simulink model "Current_torque_111"  (R2017b)
settings: Solver=ode45  StartTime=0.0  StopTime=3  MaxStep=1e-4  RelTol=1e-3  EnableMultiTasking=on
libraries: neural x38, fuzblock x6, simulink x1
(part 2 of 3)

== system Current_torque_111/CNN/Layer 5 ==
  "a{4} " : Inport  PortDimensions=5
      mask Display: e = 0.06;c1 = [120 230 180]/255;c2 = ([120 230 180]+0)/(256+128);c3 = ([120 230 180]+128)/(256+128);patch([0 1 1 0],[0 0 1 1],c1);patch([0 1 1 1-e 1-e 0+e],[0 0 1 1-e 0+e 0+e],c2);patch([0 0 1 1-e 0+e 0+e],[0 1 1 1-e 1-e 0+e],c3);plot([0 1 1 0 0],[0 0 1 1 0]);
  Delays 1 : Subsystem
      mask Display: e = 0.06;c1 = [120 150 230]/255;c2 = ([120 150 230]+0)/383;c3 = ([120 150 230]+128)/383;patch([0 1 1 0],[0 0 1 1],c1);patch([0 1 1 1-e 1-e 0+e],[0 0 1 1-e 0+e 0+e],c2);patch([0 0 1 1-e 0+e 0+e],[0 1 1 1-e 1-e 0+e],c3);plot([0 1 1 0 0],[0 0 1 1 0]);disp('0');
  "LW{5,4}" : Subsystem
      mask Display: e = 0.06;c1 = [120 150 230]/255;c2 = ([120 150 230]+0)/383;c3 = ([120 150 230]+128)/383;patch([0 1 1 0],[0 0 1 1],c1);patch([0 1 1 1-e 1-e 0+e],[0 0 1 1-e 0+e 0+e],c2);patch([0 0 1 1-e 0+e 0+e],[0 1 1 1-e 1-e 0+e],c3);plot([0 1 1 0 0],[0 0 1 1 0]);disp('W');
  "b{5}" : Constant  Value=-0.12962536607997010573711804681806825101375579833984375
      mask Display: e = 0.06;c1 = [120 150 230]/255;c2 = ([120 150 230]+0)/383;c3 = ([120 150 230]+128)/383;patch([0 1 1 0],[0 0 1 1],c1);patch([0 1 1 1-e 1-e 0+e],[0 0 1 1-e 0+e 0+e],c2);patch([0 0 1 1-e 0+e 0+e],[0 1 1 1-e 1-e 0+e],c3);plot([0 1 1 0 0],[0 0 1 1 0]);disp('b');
  netsum : Sum  Inputs=2  SaturateOnIntegerOverflow=on  InputSameDT=on  OutDataTypeStr=Inherit: Same as first input
      mask Display: e = 0.06;c1 = [120 150 230]/255;c2 = ([120 150 230]+0)/383;c3 = ([120 150 230]+128)/383;patch([0 1 1 0],[0 0 1 1],c1);patch([0 1 1 1-e 1-e 0+e],[0 0 1 1-e 0+e 0+e],c2);patch([0 0 1 1-e 0+e 0+e],[0 1 1 1-e 1-e 0+e],c3);plot([0 1 1 0 0],[0 0 1 1 0]);disp('+');
  purelin : neural/Transfer Functions/purelin
  "a{5}" : Outport  InitialOutput=0
      mask Display: e = 0.06;c1 = [120 230 180]/255;c2 = ([120 230 180]+0)/(256+128);c3 = ([120 230 180]+128)/(256+128);patch([0 1 1 0],[0 0 1 1],c1);patch([0 1 1 1-e 1-e 0+e],[0 0 1 1-e 0+e 0+e],c2);patch([0 0 1 1-e 0+e 0+e],[0 1 1 1-e 1-e 0+e],c3);plot([0 1 1 0 0],[0 0 1 1 0]);
  wires:
  purelin/1 -> "a{5}"/1
  netsum/1 -> purelin/1
  "b{5}"/1 -> netsum/2
  "LW{5,4}"/1("lz{5,4}") -> netsum/1
  Delays 1/1("pd{5,4}") -> "LW{5,4}"/1("ad{5,4}")
  "a{4} "/1 -> Delays 1/1("p{5}")

== system Current_torque_111/CNN/Process Input 1 ==
  x : Inport  PortDimensions=2
      mask Display: e = 0.06;c1 = [120 230 180]/255;c2 = ([120 230 180]+0)/(256+128);c3 = ([120 230 180]+128)/(256+128);patch([0 1 1 0],[0 0 1 1],c1);patch([0 1 1 1-e 1-e 0+e],[0 0 1 1-e 0+e 0+e],c2);patch([0 0 1 1-e 0+e 0+e],[0 1 1 1-e 1-e 0+e],c3);plot([0 1 1 0 0],[0 0 1 1 0]);
  mapminmax : neural/Processing Functions/mapminmax  xmin=[-120;1.5]  xmax=[-1;120]  ymin=-1  ymax=1
  p : Outport  PortDimensions=2
      mask Display: e = 0.06;c1 = [120 230 180]/255;c2 = ([120 230 180]+0)/(256+128);c3 = ([120 230 180]+128)/(256+128);patch([0 1 1 0],[0 0 1 1],c1);patch([0 1 1 1-e 1-e 0+e],[0 0 1 1-e 0+e 0+e],c2);patch([0 0 1 1-e 0+e 0+e],[0 1 1 1-e 1-e 0+e],c3);plot([0 1 1 0 0],[0 0 1 1 0]);
  wires:
  mapminmax/1 -> p/1
  x/1 -> mapminmax/1

== system Current_torque_111/CNN/Process Output 1 ==
  a : Inport  PortDimensions=1
      mask Display: e = 0.06;c1 = [120 230 180]/255;c2 = ([120 230 180]+0)/(256+128);c3 = ([120 230 180]+128)/(256+128);patch([0 1 1 0],[0 0 1 1],c1);patch([0 1 1 1-e 1-e 0+e],[0 0 1 1-e 0+e 0+e],c2);patch([0 0 1 1-e 0+e 0+e],[0 1 1 1-e 1-e 0+e],c3);plot([0 1 1 0 0],[0 0 1 1 0]);
  mapminmax_reverse : neural/Processing Functions/mapminmax_reverse  xmin=0.599199999999999954880536279234  xmax=104.359999999999999431565811392  ymin=-1  ymax=1
  y : Outport  PortDimensions=1
      mask Display: e = 0.06;c1 = [120 230 180]/255;c2 = ([120 230 180]+0)/(256+128);c3 = ([120 230 180]+128)/(256+128);patch([0 1 1 0],[0 0 1 1],c1);patch([0 1 1 1-e 1-e 0+e],[0 0 1 1-e 0+e 0+e],c2);patch([0 0 1 1-e 0+e 0+e],[0 1 1 1-e 1-e 0+e],c3);plot([0 1 1 0 0],[0 0 1 1 0]);
  wires:
  mapminmax_reverse/1 -> y/1
  a/1 -> mapminmax_reverse/1

== system Current_torque_111/PI Torque controller/PI-Te-iq ==
  In1 : Inport
  Integrator : Integrator  LimitOutput=on  UpperSaturationLimit=120  LowerSaturationLimit=-120
  Scope1 : Scope
  Scope3 : Scope
  Sum2 : Sum  Inputs=|++  SaturateOnIntegerOverflow=on  InputSameDT=on  OutDataTypeStr=Inherit: Same as first input
  kii : Gain  Gain=Ki  SaturateOnIntegerOverflow=on  OutDataTypeStr=Inherit: Same as input  ParamDataTypeStr=Inherit: Same as input
  kpi : Gain  Gain=Kp  SaturateOnIntegerOverflow=on  OutDataTypeStr=Inherit: Same as input  ParamDataTypeStr=Inherit: Same as input
  limit1 : Saturate  UpperLimit=120  LowerLimit=-120
  iq : Outport
  wires:
  In1/1 -> kpi/1, kii/1
  kpi/1 -> Sum2/1
  kii/1 -> Integrator/1
  Integrator/1 -> Scope1/1, Sum2/2
  Sum2/1 -> limit1/1, Scope3/1
  limit1/1 -> iq/1

== system Current_torque_111/PI current controller/PI-U-d ==
  In1 : Inport
  Integrator : Integrator  LimitOutput=on  UpperSaturationLimit=120  LowerSaturationLimit=-120
  Scope1 : Scope
  Scope3 : Scope
  Sum2 : Sum  Inputs=|++  SaturateOnIntegerOverflow=on  InputSameDT=on  OutDataTypeStr=Inherit: Same as first input
  kii : Gain  Gain=Ki  SaturateOnIntegerOverflow=on  OutDataTypeStr=Inherit: Same as input  ParamDataTypeStr=Inherit: Same as input
  kpi : Gain  Gain=Kp  SaturateOnIntegerOverflow=on  OutDataTypeStr=Inherit: Same as input  ParamDataTypeStr=Inherit: Same as input
  limit1 : Saturate  UpperLimit=120  LowerLimit=-120
  usd* : Outport
  wires:
  limit1/1 -> usd*/1
  Sum2/1 -> Scope3/1, limit1/1
  Integrator/1 -> Sum2/2, Scope1/1
  kii/1 -> Integrator/1
  kpi/1 -> Sum2/1
  In1/1 -> kii/1, kpi/1

== system Current_torque_111/PI current controller/PI-U-q ==
  In1 : Inport
  Integrator : Integrator
  Scope3 : Scope
  Sum2 : Sum  Inputs=|++  SaturateOnIntegerOverflow=on  InputSameDT=on  OutDataTypeStr=Inherit: Same as first input
  kii : Gain  Gain=Ki  SaturateOnIntegerOverflow=on  OutDataTypeStr=Inherit: Same as input  ParamDataTypeStr=Inherit: Same as input
  kpi : Gain  Gain=Kp  SaturateOnIntegerOverflow=on  OutDataTypeStr=Inherit: Same as input  ParamDataTypeStr=Inherit: Same as input
  limit2 : Saturate  UpperLimit=inf  LowerLimit=-inf
  usd* : Outport
  wires:
  limit2/1 -> usd*/1
  Sum2/1 -> Scope3/1, limit2/1
  In1/1 -> kpi/1, kii/1
  kpi/1 -> Sum2/1
  kii/1 -> Integrator/1
  Integrator/1 -> Sum2/2

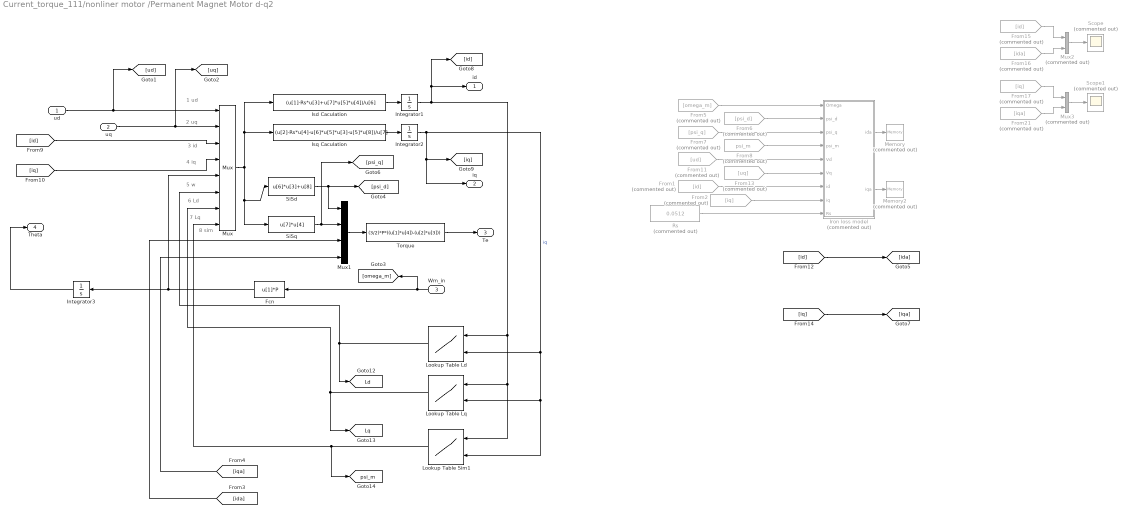
== system Current_torque_111/nonliner motor /Permanent Magnet Motor d-q2 ==
  note: 3 id
  note: 1 ud
  note: 2 uq
  note: 4 iq
  note: 5 w
  note: 6 Ld
  note: 7 Lq
  note: 8 sim
  ud : Inport
  uq : Inport  Port=2
  Wm_in : Inport  Port=3
  Fcn : Fcn  Expr=u[1]*P
  From1 : From  Commented=on  GotoTag=id
  From11 : From  Commented=on  GotoTag=ud
  From13 : From  Commented=on  GotoTag=uq
  From15 : From  Commented=on  GotoTag=id
  From16 : From  Commented=on  GotoTag=ida
  From17 : From  Commented=on  GotoTag=iq
  From2 : From  Commented=on  GotoTag=iq
  From21 : From  Commented=on  GotoTag=iqa
  From5 : From  Commented=on  GotoTag=omega_m
  From6 : From  Commented=on  GotoTag=psi_d
  From7 : From  Commented=on  GotoTag=psi_q
  From8 : From  Commented=on  GotoTag=psi_m  TagVisibility=global
  Integrator1 : Integrator
  Integrator2 : Integrator
  Integrator3 : Integrator
  Iron loss model : Subsystem  Commented=on
  Isd Caculation : Fcn  Expr=(u[1]-Rs*u[3]+u[7]*u[5]*u[4])/u[6]
  Isq Caculation : Fcn  Expr=(u[2]-Rs*u[4]-u[6]*u[5]*u[3]-u[5]*u[8])/u[7]
  Lookup Table Ld : Lookup2D  RowIndex=|  ColumnIndex=|  Table=1e-3*[[0.843,0.842,0.841,0.835,0.822,0.812,0.791,0.763,0.733,0.707,0.683,0.661,0.639];[0.848,0.847,0.846,0.840,0.831,0.814,0.786,0.754,0.723,0.695,0.674,0.651,0.631];[0.852,0.851,0.848,0.844,0.836,0.813,0.777,0.740,0.705,0.682,0.658,0.636,0.618];[0.858,0.857,0.856,0.848,0.831,0.806,0.763,0.727,0.695,0.664,0.643,0.620,0.602];[0.864,0.863,0.860,0.852,0.829,0.796,0.758,0.715,0.682,0.655,0.629,0.607,0.586];[0.870,0.867,0.863,0.850,0.820,0.783,0.748,0.712,0.677,0.650,0.624,0.600,0.580];[0.882,0.875,0.868,0.848,0.808,0.770,0.735,0.707,0.682,0.653,0.621,0.602,0.576];[0.892,0.889,0.873,0.835,0.796,0.757,0.723,0.701,0.678,0.653,0.632,0.603,0.575];[0.902,0.896,0.869,0.819,0.773,0.741,0.712,0.683,0.663,0.646,0.626,0.604,0.584];[0.906,0.892,0.843,0.786,0.750,0.713,0.691,0.662,0.643,0.629,0.611,0.595,0.576];[0.891,0.860,0.798,0.747,0.704,0.685,0.664,0.640,0.615,0.602,0.596,0.576,0.566];[0.838,0.800,0.749,0.707,0.670,0.653,0.628,0.613,0.588,0.576,0.562,0.558,0.546];[0.733,0.700,0.667,0.636,0.612,0.605,0.594,0.579,0.564,0.544,0.529,0.521,0.517]]
      RowIndex=|
      | [-119.9923
      | -109.9929
      | -99.9936
      | -89.9943
      | -79.9949
      | -69.9955
      | -59.9962
      | -49.9968
      | -39.9974
      | -29.9981
      | -19.9987
      | -9.9994
      | 0]
      ColumnIndex=|
      | [0.0000
      | 9.9613
      | 20.0042
      | 29.9654
      | 40.0083
      | 49.9696
      | 60.0125
      | 69.9738
      | 80.0167
      | 89.8146
      | 99.6126
      | 110.2270
      | 120.0250]
  Lookup Table Lq : Lookup2D  RowIndex=|  ColumnIndex=|  Table=1e-3*[[2.7,2.65,2.62,2.45,2.3,2.23,2.1,1.85,1.74,1.61,1.5,1.43,1.33];[2.75,2.7,2.65,2.46,2.31,2.22,2.08,1.84,1.73,1.6,1.49,1.42,1.32];[2.8,2.75,2.7,2.47,2.32,2.21,2.05,1.83,1.72,1.59,1.48,1.4,1.31];[2.9,2.8,2.72,2.48,2.33,2.2,2.02,1.82,1.71,1.58,1.47,1.37,1.3];[2.95,2.85,2.74,2.49,2.34,2.15,2,1.81,1.7,1.57,1.46,1.35,1.29];[3,2.9,2.77,2.5,2.33,2.14,1.95,1.8,1.67,1.56,1.45,1.34,1.28];[3.1,2.95,2.79,2.51,2.32,2.13,1.92,1.79,1.65,1.55,1.44,1.33,1.27];[3.2,3,2.8,2.52,2.3,2.1,1.9,1.75,1.63,1.54,1.43,1.32,1.26];[3.3,3.07,2.78,2.5,2.25,2,1.85,1.72,1.6,1.53,1.4,1.31,1.25];[3.37,3.1,2.75,2.45,2.2,1.99,1.82,1.7,1.55,1.48,1.38,1.3,1.24];[3.4,3.05,2.7,2.4,2.15,1.98,1.8,1.68,1.52,1.46,1.36,1.28,1.23];[3.35,3.02,2.65,2.35,2.1,1.95,1.75,1.65,1.51,1.44,1.35,1.25,1.22];[3.3,3,2.6,2.3,2,1.9,1.7,1.6,1.5,1.4,1.3,1.22,1.2]]
      RowIndex=|
      | [-119.9923
      | -109.9929
      | -99.9936
      | -89.9943
      | -79.9949
      | -69.9955
      | -59.9962
      | -49.9968
      | -39.9974
      | -29.9981
      | -19.9987
      | -9.9994
      | 0]
      ColumnIndex=|
      | [0.0000
      | 9.9613
      | 20.0042
      | 29.9654
      | 40.0083
      | 49.9696
      | 60.0125
      | 69.9738
      | 80.0167
      | 89.8146
      | 99.6126
      | 110.2270
      | 120.0250]
  Lookup Table Sim1 : Lookup2D  RowIndex=|  ColumnIndex=|  Table=1e-3*[[129.6,128.4,127.5,126.5,125.5,124,123,121,119.8,118.2,116.5,114.2,110.3];[129.7,127.2,126.2,125,124,123,122,120,119,117.1,115,112.2,106.4];[130,126.2,125,123.5,122,121,120,118,116,114.7,112,110.5,104.1];[130.4,126.6,123.5,122.2,121,118,117,115,113,112,110,108,101.8];[130.8,127.6,123,120.5,118.9,116.5,113,111,110,108.8,107.5,106,100.4];[131.2,128.2,125.1,118.8,116.3,115,111.6,110,108.9,107,105,104,98.1];[131.9,130,127,118.1,115.0,113.4,110,109,107,104.2,102.8,101.2,96.7];[132.4,130.5,128,119.4,114,113,109.5,108,106,102.9,101.6,100.5,95.1];[132.8,130.6,128.7,120.5,114.5,113.5,110.8,107.5,105.6,101.7,100.5,98.8,94.5];[132.9,130.2,127.9,121,115.5,112.7,110.5,108.5,106.5,103.2,101.5,98.9,92.7];[132.2,129.9,125.9,121.3,115.9,111.5,109.4,107.8,107,102.7,101,97.5,91.1];[131.5,129.0,125.6,120.7,115.3,110.7,109,108,106.6,102.6,99.7,95.9,88.7];[130.8,128.6,124.6,120.5,117.4,111.4,110,109,107.5,103.1,100.4,96.5,88.6]]
      RowIndex=|
      | [-119.9923
      | -109.9929
      | -99.9936
      | -89.9943
      | -79.9949
      | -69.9955
      | -59.9962
      | -49.9968
      | -39.9974
      | -29.9981
      | -19.9987
      | -9.9994
      | 0]
      ColumnIndex=|
      | [0.0000
      | 9.9613
      | 20.0042
      | 29.9654
      | 40.0083
      | 49.9696
      | 60.0125
      | 69.9738
      | 80.0167
      | 89.8146
      | 99.6126
      | 110.2270
      | 120.0250]
  Memory : Memory  Commented=on
  Memory2 : Memory  Commented=on
  Mux : Mux  Inputs=8
  Mux1 : Mux
  Mux2 : Mux  Commented=on  Inputs=2
  Mux3 : Mux  Commented=on  Inputs=2
  Rs : Constant  Commented=on  Value=0.0512
  Scope : Scope  Commented=on
  Scope1 : Scope  Commented=on
  SiSd : Fcn  Expr=u[6]*u[3]+u[8]
  SiSq : Fcn  Expr=u[7]*u[4]
  Torque : Fcn  Expr=(3/2)*P*((u[1]*u[4])-(u[2]*u[3]))
  id : Outport
  iq : Outport  Port=2
  Te : Outport  Port=3
  Theta : Outport  Port=4
  tag scope: Ld=global, Lq=global, psi_m=global
  wires:
  Mux/1 -> Isq Caculation/1, Isd Caculation/1, SiSq/1, SiSd/1
  Integrator2/1 -> iq/1, [iq], Lookup Table Ld/2, Lookup Table Lq/2, Lookup Table Sim1/2  "iq"
  Fcn/1 -> Mux/5, Integrator3/1
  Integrator3/1 -> Theta/1
  Mux1/1 -> Torque/1
  Torque/1 -> Te/1
  SiSd/1 -> [psi_d], Mux1/1
  SiSq/1 -> [psi_q], Mux1/2
  Wm_in/1 -> [omega_m], Fcn/1
  From5/1 -> Iron loss model/1(Omega)
  Iron loss model/1(ida) -> Memory/1
  Iron loss model/2(iqa) -> Memory2/1
  Rs/1 -> Iron loss model/9(Rs)
  Isd Caculation/1 -> Integrator1/1
  Isq Caculation/1 -> Integrator2/1
  Lookup Table Sim1/1 -> [psi_m], Mux/8
  Lookup Table Lq/1 -> [Lq], Mux/7
  Lookup Table Ld/1 -> [Ld], Mux/6
  [ida] -> Mux1/3
  [iqa] -> Mux1/4
  From1/1 -> Iron loss model/7(id)
  ud/1 -> [ud], Mux/1
  uq/1 -> [uq], Mux/2
  From2/1 -> Iron loss model/8(iq)
  Integrator1/1 -> id/1, [id], Lookup Table Sim1/1, Lookup Table Lq/1, Lookup Table Ld/1
  [id] -> Mux/3
  [iq] -> Mux/4
  From6/1 -> Iron loss model/2(psi_d)
  From7/1 -> Iron loss model/3(psi_q)
  From8/1 -> Iron loss model/4(psi_m)
  Mux2/1 -> Scope/1
  From15/1 -> Mux2/1
  From16/1 -> Mux2/2
  Mux3/1 -> Scope1/1
  From17/1 -> Mux3/1
  From21/1 -> Mux3/2
  From11/1 -> Iron loss model/5(Vd)
  From13/1 -> Iron loss model/6(Vq)
  [id] -> [ida]
  [iq] -> [iqa]

== system Current_torque_111/CNN/Layer 1/Delays 1 ==
  "p{1}" : Inport  PortDimensions=2
      mask Display: e = 0.06;c1 = [120 230 180]/255;c2 = ([120 230 180]+0)/(256+128);c3 = ([120 230 180]+128)/(256+128);patch([0 1 1 0],[0 0 1 1],c1);patch([0 1 1 1-e 1-e 0+e],[0 0 1 1-e 0+e 0+e],c2);patch([0 0 1 1-e 0+e 0+e],[0 1 1 1-e 1-e 0+e],c3);plot([0 1 1 0 0],[0 0 1 1 0]);
  mux : Mux  Inputs=1
      mask Display: e = 0.06;c1 = [120 150 230]/255;c2 = ([120 150 230]+0)/383;c3 = ([120 150 230]+128)/383;patch([0 1 1 0],[0 0 1 1],c1);patch([0 1 1 1-e 1-e 0+e],[0 0 1 1-e 0+e 0+e],c2);patch([0 0 1 1-e 0+e 0+e],[0 1 1 1-e 1-e 0+e],c3);plot([0 1 1 0 0],[0 0 1 1 0]);disp('Mux')
  "pd{1,1}" : Outport
      mask Display: e = 0.06;c1 = [120 230 180]/255;c2 = ([120 230 180]+0)/(256+128);c3 = ([120 230 180]+128)/(256+128);patch([0 1 1 0],[0 0 1 1],c1);patch([0 1 1 1-e 1-e 0+e],[0 0 1 1-e 0+e 0+e],c2);patch([0 0 1 1-e 0+e 0+e],[0 1 1 1-e 1-e 0+e],c3);plot([0 1 1 0 0],[0 0 1 1 0]);
  wires:
  mux/1 -> "pd{1,1}"/1
  "p{1}"/1 -> mux/1

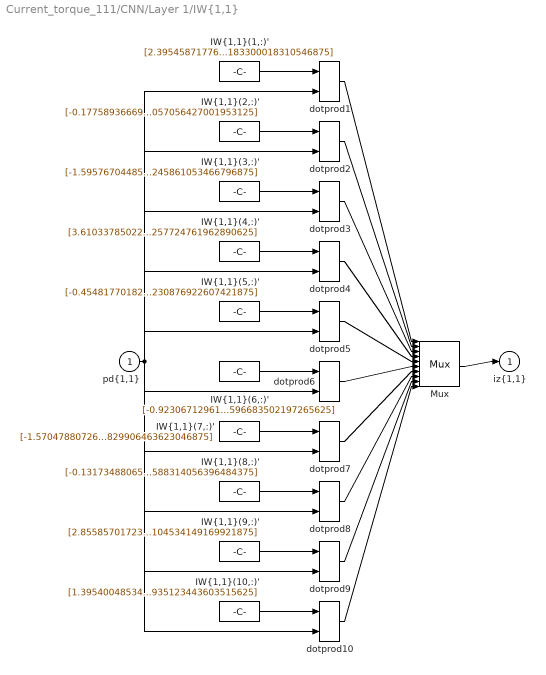
== system Current_torque_111/CNN/Layer 1/IW{1,1} ==
  "pd{1,1}" : Inport  PortDimensions=2
      mask Display: e = 0.06;c1 = [120 230 180]/255;c2 = ([120 230 180]+0)/(256+128);c3 = ([120 230 180]+128)/(256+128);patch([0 1 1 0],[0 0 1 1],c1);patch([0 1 1 1-e 1-e 0+e],[0 0 1 1-e 0+e 0+e],c2);patch([0 0 1 1-e 0+e 0+e],[0 1 1 1-e 1-e 0+e],c3);plot([0 1 1 0 0],[0 0 1 1 0]);
  "IW{1,1}(1,:)'" : Constant  Value=[2.395458717766983713914896725327707827091217041015625;-4.07814613796772373888188667478971183300018310546875]
      mask Display: e = 0.06;c1 = [120 150 230]/255;c2 = ([120 150 230]+0)/383;c3 = ([120 150 230]+128)/383;patch([0 1 1 0],[0 0 1 1],c1);patch([0 1 1 1-e 1-e 0+e],[0 0 1 1-e 0+e 0+e],c2);patch([0 0 1 1-e 0+e 0+e],[0 1 1 1-e 1-e 0+e],c3);plot([0 1 1 0 0],[0 0 1 1 0]);disp('Weights');
  "IW{1,1}(10,:)'" : Constant  Value=[1.395400485348682995123681394034065306186676025390625;2.747381883526897272673750194371677935123443603515625]
      mask Display: e = 0.06;c1 = [120 150 230]/255;c2 = ([120 150 230]+0)/383;c3 = ([120 150 230]+128)/383;patch([0 1 1 0],[0 0 1 1],c1);patch([0 1 1 1-e 1-e 0+e],[0 0 1 1-e 0+e 0+e],c2);patch([0 0 1 1-e 0+e 0+e],[0 1 1 1-e 1-e 0+e],c3);plot([0 1 1 0 0],[0 0 1 1 0]);disp('Weights');
  "IW{1,1}(2,:)'" : Constant  Value=[-0.17758936669711145039940447531989775598049163818359375;3.962517618146396802814024340477772057056427001953125]
      mask Display: e = 0.06;c1 = [120 150 230]/255;c2 = ([120 150 230]+0)/383;c3 = ([120 150 230]+128)/383;patch([0 1 1 0],[0 0 1 1],c1);patch([0 1 1 1-e 1-e 0+e],[0 0 1 1-e 0+e 0+e],c2);patch([0 0 1 1-e 0+e 0+e],[0 1 1 1-e 1-e 0+e],c3);plot([0 1 1 0 0],[0 0 1 1 0]);disp('Weights');
  "IW{1,1}(3,:)'" : Constant  Value=[-1.5957670448510923311147280401200987398624420166015625;4.255626203502782090026812511496245861053466796875]
      mask Display: e = 0.06;c1 = [120 150 230]/255;c2 = ([120 150 230]+0)/383;c3 = ([120 150 230]+128)/383;patch([0 1 1 0],[0 0 1 1],c1);patch([0 1 1 1-e 1-e 0+e],[0 0 1 1-e 0+e 0+e],c2);patch([0 0 1 1-e 0+e 0+e],[0 1 1 1-e 1-e 0+e],c3);plot([0 1 1 0 0],[0 0 1 1 0]);disp('Weights');
  "IW{1,1}(4,:)'" : Constant  Value=[3.610337850220468158823905469034798443317413330078125;-0.94293319089329319382386529468931257724761962890625]
      mask Display: e = 0.06;c1 = [120 150 230]/255;c2 = ([120 150 230]+0)/383;c3 = ([120 150 230]+128)/383;patch([0 1 1 0],[0 0 1 1],c1);patch([0 1 1 1-e 1-e 0+e],[0 0 1 1-e 0+e 0+e],c2);patch([0 0 1 1-e 0+e 0+e],[0 1 1 1-e 1-e 0+e],c3);plot([0 1 1 0 0],[0 0 1 1 0]);disp('Weights');
  "IW{1,1}(5,:)'" : Constant  Value=[-0.45481770182663827650770826949155889451503753662109375;4.51560678784560831644512290949933230876922607421875]
      mask Display: e = 0.06;c1 = [120 150 230]/255;c2 = ([120 150 230]+0)/383;c3 = ([120 150 230]+128)/383;patch([0 1 1 0],[0 0 1 1],c1);patch([0 1 1 1-e 1-e 0+e],[0 0 1 1-e 0+e 0+e],c2);patch([0 0 1 1-e 0+e 0+e],[0 1 1 1-e 1-e 0+e],c3);plot([0 1 1 0 0],[0 0 1 1 0]);disp('Weights');
  "IW{1,1}(6,:)'" : Constant  Value=[-0.9230671296193471153657128525082953274250030517578125;-0.8434159316909506376447325237677432596683502197265625]
      mask Display: e = 0.06;c1 = [120 150 230]/255;c2 = ([120 150 230]+0)/383;c3 = ([120 150 230]+128)/383;patch([0 1 1 0],[0 0 1 1],c1);patch([0 1 1 1-e 1-e 0+e],[0 0 1 1-e 0+e 0+e],c2);patch([0 0 1 1-e 0+e 0+e],[0 1 1 1-e 1-e 0+e],c3);plot([0 1 1 0 0],[0 0 1 1 0]);disp('Weights');
  "IW{1,1}(7,:)'" : Constant  Value=[-1.57047880726612021362598170526325702667236328125;-1.6323780385539687909357553508016280829906463623046875]
      mask Display: e = 0.06;c1 = [120 150 230]/255;c2 = ([120 150 230]+0)/383;c3 = ([120 150 230]+128)/383;patch([0 1 1 0],[0 0 1 1],c1);patch([0 1 1 1-e 1-e 0+e],[0 0 1 1-e 0+e 0+e],c2);patch([0 0 1 1-e 0+e 0+e],[0 1 1 1-e 1-e 0+e],c3);plot([0 1 1 0 0],[0 0 1 1 0]);disp('Weights');
  "IW{1,1}(8,:)'" : Constant  Value=[-0.131734880659383157830433219714905135333538055419921875;1.0191892430950291181801503626047633588314056396484375]
      mask Display: e = 0.06;c1 = [120 150 230]/255;c2 = ([120 150 230]+0)/383;c3 = ([120 150 230]+128)/383;patch([0 1 1 0],[0 0 1 1],c1);patch([0 1 1 1-e 1-e 0+e],[0 0 1 1-e 0+e 0+e],c2);patch([0 0 1 1-e 0+e 0+e],[0 1 1 1-e 1-e 0+e],c3);plot([0 1 1 0 0],[0 0 1 1 0]);disp('Weights');
  "IW{1,1}(9,:)'" : Constant  Value=[2.855857017238718764673421901534311473369598388671875;3.21481337784656329148447184707038104534149169921875]
      mask Display: e = 0.06;c1 = [120 150 230]/255;c2 = ([120 150 230]+0)/383;c3 = ([120 150 230]+128)/383;patch([0 1 1 0],[0 0 1 1],c1);patch([0 1 1 1-e 1-e 0+e],[0 0 1 1-e 0+e 0+e],c2);patch([0 0 1 1-e 0+e 0+e],[0 1 1 1-e 1-e 0+e],c3);plot([0 1 1 0 0],[0 0 1 1 0]);disp('Weights');
  Mux : Mux  Inputs=10
      mask Display: e = 0.06;c1 = [120 150 230]/255;c2 = ([120 150 230]+0)/383;c3 = ([120 150 230]+128)/383;patch([0 1 1 0],[0 0 1 1],c1);patch([0 1 1 1-e 1-e 0+e],[0 0 1 1-e 0+e 0+e],c2);patch([0 0 1 1-e 0+e 0+e],[0 1 1 1-e 1-e 0+e],c3);plot([0 1 1 0 0],[0 0 1 1 0]);disp('Mux');
  dotprod{1..10} (10 alike) : neural/Weight Functions/dotprod
  "iz{1,1}" : Outport
      mask Display: e = 0.06;c1 = [120 230 180]/255;c2 = ([120 230 180]+0)/(256+128);c3 = ([120 230 180]+128)/(256+128);patch([0 1 1 0],[0 0 1 1],c1);patch([0 1 1 1-e 1-e 0+e],[0 0 1 1-e 0+e 0+e],c2);patch([0 0 1 1-e 0+e 0+e],[0 1 1 1-e 1-e 0+e],c3);plot([0 1 1 0 0],[0 0 1 1 0]);
  wires:
  Mux/1 -> "iz{1,1}"/1
  dotprod10/1 -> Mux/10
  "IW{1,1}(10,:)'"/1 -> dotprod10/1
  dotprod9/1 -> Mux/9
  "IW{1,1}(9,:)'"/1 -> dotprod9/1
  dotprod8/1 -> Mux/8
  "IW{1,1}(8,:)'"/1 -> dotprod8/1
  dotprod7/1 -> Mux/7
  "IW{1,1}(7,:)'"/1 -> dotprod7/1
  dotprod6/1 -> Mux/6
  "IW{1,1}(6,:)'"/1 -> dotprod6/1
  dotprod5/1 -> Mux/5
  "IW{1,1}(5,:)'"/1 -> dotprod5/1
  dotprod4/1 -> Mux/4
  "IW{1,1}(4,:)'"/1 -> dotprod4/1
  dotprod3/1 -> Mux/3
  "IW{1,1}(3,:)'"/1 -> dotprod3/1
  dotprod2/1 -> Mux/2
  "IW{1,1}(2,:)'"/1 -> dotprod2/1
  dotprod1/1 -> Mux/1
  "pd{1,1}"/1 -> dotprod10/2, dotprod9/2, dotprod8/2, dotprod7/2, dotprod6/2, dotprod5/2, dotprod4/2, dotprod3/2, dotprod2/2, dotprod1/2
  "IW{1,1}(1,:)'"/1 -> dotprod1/1

== system Current_torque_111/CNN/Layer 2/Delays 1 ==
  "p{2}" : Inport  PortDimensions=10
      mask Display: e = 0.06;c1 = [120 230 180]/255;c2 = ([120 230 180]+0)/(256+128);c3 = ([120 230 180]+128)/(256+128);patch([0 1 1 0],[0 0 1 1],c1);patch([0 1 1 1-e 1-e 0+e],[0 0 1 1-e 0+e 0+e],c2);patch([0 0 1 1-e 0+e 0+e],[0 1 1 1-e 1-e 0+e],c3);plot([0 1 1 0 0],[0 0 1 1 0]);
  mux : Mux  Inputs=1
      mask Display: e = 0.06;c1 = [120 150 230]/255;c2 = ([120 150 230]+0)/383;c3 = ([120 150 230]+128)/383;patch([0 1 1 0],[0 0 1 1],c1);patch([0 1 1 1-e 1-e 0+e],[0 0 1 1-e 0+e 0+e],c2);patch([0 0 1 1-e 0+e 0+e],[0 1 1 1-e 1-e 0+e],c3);plot([0 1 1 0 0],[0 0 1 1 0]);disp('Mux')
  "pd{2,1}" : Outport
      mask Display: e = 0.06;c1 = [120 230 180]/255;c2 = ([120 230 180]+0)/(256+128);c3 = ([120 230 180]+128)/(256+128);patch([0 1 1 0],[0 0 1 1],c1);patch([0 1 1 1-e 1-e 0+e],[0 0 1 1-e 0+e 0+e],c2);patch([0 0 1 1-e 0+e 0+e],[0 1 1 1-e 1-e 0+e],c3);plot([0 1 1 0 0],[0 0 1 1 0]);
  wires:
  mux/1 -> "pd{2,1}"/1
  "p{2}"/1 -> mux/1

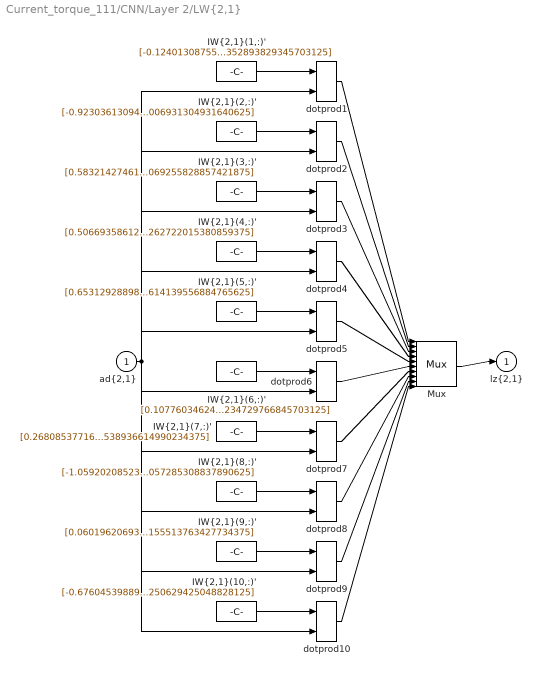
== system Current_torque_111/CNN/Layer 2/LW{2,1} ==
  "ad{2,1}" : Inport  PortDimensions=10
      mask Display: e = 0.06;c1 = [120 230 180]/255;c2 = ([120 230 180]+0)/(256+128);c3 = ([120 230 180]+128)/(256+128);patch([0 1 1 0],[0 0 1 1],c1);patch([0 1 1 1-e 1-e 0+e],[0 0 1 1-e 0+e 0+e],c2);patch([0 0 1 1-e 0+e 0+e],[0 1 1 1-e 1-e 0+e],c3);plot([0 1 1 0 0],[0 0 1 1 0]);
  "IW{2,1}(1,:)'" : Constant  Value=[-0.12401308755404370776087574768098420463502407073974609375;-0.06639906464640925320974673695673118345439434051513671875;-0.331999175988151318250629628892056643962860107421875;0.1184071623869516753924102658857009373605251312255859375;0.005795490518349225884942033104607617133297026157379150390625;0.639113863758823175231782443006522953510284423828125;-1.1334791361583314017735801826347596943378448486328125;-1.208761307275062701904744244529865682125091552734375;-0.1624777703301522879808516108823823742568492889404296875;-0.44594068348848470151324363541789352893829345703125]
      mask Display: e = 0.06;c1 = [120 150 230]/255;c2 = ([120 150 230]+0)/383;c3 = ([120 150 230]+128)/383;patch([0 1 1 0],[0 0 1 1],c1);patch([0 1 1 1-e 1-e 0+e],[0 0 1 1-e 0+e 0+e],c2);patch([0 0 1 1-e 0+e 0+e],[0 1 1 1-e 1-e 0+e],c3);plot([0 1 1 0 0],[0 0 1 1 0]);disp('weights');
  "IW{2,1}(10,:)'" : Constant  Value=[-0.67604539889036352473539182028616778552532196044921875;-0.52177633078488394602345579187385737895965576171875;0.86237455739704282908775212490581907331943511962890625;-0.072307556694448660294938235892914235591888427734375;-0.74284278863900399247910399935790337622165679931640625;0.10972241684503257486138494414262822829186916351318359375;-0.2381257386608559567520160271669737994670867919921875;-0.50307529909243664523188499515526928007602691650390625;0.0624718902209848991891050218328018672764301300048828125;0.1903884224866004004628194934412022121250629425048828125]
      mask Display: e = 0.06;c1 = [120 150 230]/255;c2 = ([120 150 230]+0)/383;c3 = ([120 150 230]+128)/383;patch([0 1 1 0],[0 0 1 1],c1);patch([0 1 1 1-e 1-e 0+e],[0 0 1 1-e 0+e 0+e],c2);patch([0 0 1 1-e 0+e 0+e],[0 1 1 1-e 1-e 0+e],c3);plot([0 1 1 0 0],[0 0 1 1 0]);disp('weights');
  "IW{2,1}(2,:)'" : Constant  Value=[-0.92303613094291947493985617256839759647846221923828125;-0.88438291504655175412352718922193162143230438232421875;-0.272482241344422337903097286471165716648101806640625;1.0621320297256009457242953430977649986743927001953125;0.1959660851108216694793640044736093841493129730224609375;1.85711136011126587419539646361954510211944580078125;-0.079652478792025693810074926659581251442432403564453125;-0.61483819400785433284539749365649186074733734130859375;0.178674361953623239696042901414330117404460906982421875;-1.4613200004086766004007813535281457006931304931640625]
      mask Display: e = 0.06;c1 = [120 150 230]/255;c2 = ([120 150 230]+0)/383;c3 = ([120 150 230]+128)/383;patch([0 1 1 0],[0 0 1 1],c1);patch([0 1 1 1-e 1-e 0+e],[0 0 1 1-e 0+e 0+e],c2);patch([0 0 1 1-e 0+e 0+e],[0 1 1 1-e 1-e 0+e],c3);plot([0 1 1 0 0],[0 0 1 1 0]);disp('weights');
  "IW{2,1}(3,:)'" : Constant  Value=[0.5832142746149935330635116770281456410884857177734375;1.98094269114918031249317209585569798946380615234375;0.401369006184528809288991624271147884428501129150390625;-0.64034646465361688694173381009022705256938934326171875;-1.616328016876521278533118675113655626773834228515625;2.0987053810323690328232260071672499179840087890625;1.405321720446348177091522302362136542797088623046875;-0.15783228894274781151096931353094987571239471435546875;2.171719551176290341487629120820201933383941650390625;0.30096199314076066411161036739940755069255828857421875]
      mask Display: e = 0.06;c1 = [120 150 230]/255;c2 = ([120 150 230]+0)/383;c3 = ([120 150 230]+128)/383;patch([0 1 1 0],[0 0 1 1],c1);patch([0 1 1 1-e 1-e 0+e],[0 0 1 1-e 0+e 0+e],c2);patch([0 0 1 1-e 0+e 0+e],[0 1 1 1-e 1-e 0+e],c3);plot([0 1 1 0 0],[0 0 1 1 0]);disp('weights');
  "IW{2,1}(4,:)'" : Constant  Value=[0.5066935861204771018861947595723904669284820556640625;-2.0366462355801786543452180922031402587890625;-0.24095322956472264852578746285871602594852447509765625;0.08709958710505409651414510108224931173026561737060546875;0.0793317700008100146202849600740591995418071746826171875;-1.337515914245819725891806228901259601116180419921875;-0.24938029110327575299521640772582031786441802978515625;2.925637031337599669456039919168688356876373291015625;-1.0388436354915329129511292194365523755550384521484375;0.346665651488343440345119006451568566262722015380859375]
      mask Display: e = 0.06;c1 = [120 150 230]/255;c2 = ([120 150 230]+0)/383;c3 = ([120 150 230]+128)/383;patch([0 1 1 0],[0 0 1 1],c1);patch([0 1 1 1-e 1-e 0+e],[0 0 1 1-e 0+e 0+e],c2);patch([0 0 1 1-e 0+e 0+e],[0 1 1 1-e 1-e 0+e],c3);plot([0 1 1 0 0],[0 0 1 1 0]);disp('weights');
  "IW{2,1}(5,:)'" : Constant  Value=[0.6531292889867377216006616436061449348926544189453125;1.1309824413983042834530579057172872126102447509765625;-0.0031624433188201235382652765082411860930733382701873779296875;-0.47127129335165196533097287101554684340953826904296875;-0.805945610564921199880927815684117376804351806640625;0.3317054283272129477921907891868613660335540771484375;0.85918761082891415004070267968927510082721710205078125;0.2415276295807365081191875333388452418148517608642578125;-1.142588066335395335926250481861643493175506591796875;-0.0958359386935540291663215839434997178614139556884765625]
      mask Display: e = 0.06;c1 = [120 150 230]/255;c2 = ([120 150 230]+0)/383;c3 = ([120 150 230]+128)/383;patch([0 1 1 0],[0 0 1 1],c1);patch([0 1 1 1-e 1-e 0+e],[0 0 1 1-e 0+e 0+e],c2);patch([0 0 1 1-e 0+e 0+e],[0 1 1 1-e 1-e 0+e],c3);plot([0 1 1 0 0],[0 0 1 1 0]);disp('weights');
  "IW{2,1}(6,:)'" : Constant  Value=[0.107760346247176952427793139577261172235012054443359375;0.33431863558241314837715663088602013885974884033203125;0.2227067049336723114638658671537996269762516021728515625;0.0286998597777812398945673777461706777103245258331298828125;0.45153163612632152279502406599931418895721435546875;-0.60888670996221228026712424252764321863651275634765625;0.7337049028534698980053008199320174753665924072265625;-0.79801962851422292288816606742329895496368408203125;0.13794470820666260291176286045811139047145843505859375;-0.118096456714982533942048803510260768234729766845703125]
      mask Display: e = 0.06;c1 = [120 150 230]/255;c2 = ([120 150 230]+0)/383;c3 = ([120 150 230]+128)/383;patch([0 1 1 0],[0 0 1 1],c1);patch([0 1 1 1-e 1-e 0+e],[0 0 1 1-e 0+e 0+e],c2);patch([0 0 1 1-e 0+e 0+e],[0 1 1 1-e 1-e 0+e],c3);plot([0 1 1 0 0],[0 0 1 1 0]);disp('weights');
  "IW{2,1}(7,:)'" : Constant  Value=[0.2680853771662088380622890326776541769504547119140625;-0.59041595751116482393427986608003266155719757080078125;-0.1364877001110826049146140803713933564722537994384765625;0.60441910259129916216380706828203983604907989501953125;0.113646717194798296812763283014646731317043304443359375;-2.557346164050288361835328032611869275569915771484375;1.234985142242049693805938659352250397205352783203125;-2.023010760419541753662997507490217685699462890625;0.31089966125333712287925891359918750822544097900390625;-1.520683529651600363052921238704584538936614990234375]
      mask Display: e = 0.06;c1 = [120 150 230]/255;c2 = ([120 150 230]+0)/383;c3 = ([120 150 230]+128)/383;patch([0 1 1 0],[0 0 1 1],c1);patch([0 1 1 1-e 1-e 0+e],[0 0 1 1-e 0+e 0+e],c2);patch([0 0 1 1-e 0+e 0+e],[0 1 1 1-e 1-e 0+e],c3);plot([0 1 1 0 0],[0 0 1 1 0]);disp('weights');
  "IW{2,1}(8,:)'" : Constant  Value=[-1.0592020852348842385737270888057537376880645751953125;-0.70553511890070452761136721164803020656108856201171875;-0.2304167140004869107627882840461097657680511474609375;-0.2093566946482075252777832474748720414936542510986328125;1.84247523873457108578577390289865434169769287109375;-1.0102323323615085559623594235745258629322052001953125;-0.0251643586501676431999019456497990177012979984283447265625;0.876004509639025652489863205119036138057708740234375;0.33331024216624083322813021368347108364105224609375;0.08997643424951073942708035247051157057285308837890625]
      mask Display: e = 0.06;c1 = [120 150 230]/255;c2 = ([120 150 230]+0)/383;c3 = ([120 150 230]+128)/383;patch([0 1 1 0],[0 0 1 1],c1);patch([0 1 1 1-e 1-e 0+e],[0 0 1 1-e 0+e 0+e],c2);patch([0 0 1 1-e 0+e 0+e],[0 1 1 1-e 1-e 0+e],c3);plot([0 1 1 0 0],[0 0 1 1 0]);disp('weights');
  "IW{2,1}(9,:)'" : Constant  Value=[0.0601962069314285475041259587669628672301769256591796875;0.337398227790713323148708013832219876348972320556640625;0.43957826822111545350679762123036198318004608154296875;-0.0850323950437066600205326949435402639210224151611328125;0.54107535708049836475908023203373886644840240478515625;-1.4421251198678228799820999483927153050899505615234375;1.0443604445776439870741114646079950034618377685546875;-3.047258949964206209415351622737944126129150390625;0.262941439331294934955707276458269916474819183349609375;-0.14370354244001981580680649130954407155513763427734375]
      mask Display: e = 0.06;c1 = [120 150 230]/255;c2 = ([120 150 230]+0)/383;c3 = ([120 150 230]+128)/383;patch([0 1 1 0],[0 0 1 1],c1);patch([0 1 1 1-e 1-e 0+e],[0 0 1 1-e 0+e 0+e],c2);patch([0 0 1 1-e 0+e 0+e],[0 1 1 1-e 1-e 0+e],c3);plot([0 1 1 0 0],[0 0 1 1 0]);disp('weights');
  Mux : Mux  Inputs=10
      mask Display: e = 0.06;c1 = [120 150 230]/255;c2 = ([120 150 230]+0)/383;c3 = ([120 150 230]+128)/383;patch([0 1 1 0],[0 0 1 1],c1);patch([0 1 1 1-e 1-e 0+e],[0 0 1 1-e 0+e 0+e],c2);patch([0 0 1 1-e 0+e 0+e],[0 1 1 1-e 1-e 0+e],c3);plot([0 1 1 0 0],[0 0 1 1 0]);disp('Mux');
  dotprod{1..10} (10 alike) : neural/Weight Functions/dotprod
  "lz{2,1}" : Outport
      mask Display: e = 0.06;c1 = [120 230 180]/255;c2 = ([120 230 180]+0)/(256+128);c3 = ([120 230 180]+128)/(256+128);patch([0 1 1 0],[0 0 1 1],c1);patch([0 1 1 1-e 1-e 0+e],[0 0 1 1-e 0+e 0+e],c2);patch([0 0 1 1-e 0+e 0+e],[0 1 1 1-e 1-e 0+e],c3);plot([0 1 1 0 0],[0 0 1 1 0]);
  wires:
  Mux/1 -> "lz{2,1}"/1
  dotprod10/1 -> Mux/10
  "IW{2,1}(10,:)'"/1 -> dotprod10/1
  dotprod9/1 -> Mux/9
  "IW{2,1}(9,:)'"/1 -> dotprod9/1
  dotprod8/1 -> Mux/8
  "IW{2,1}(8,:)'"/1 -> dotprod8/1
  dotprod7/1 -> Mux/7
  "IW{2,1}(7,:)'"/1 -> dotprod7/1
  dotprod6/1 -> Mux/6
  "IW{2,1}(6,:)'"/1 -> dotprod6/1
  dotprod5/1 -> Mux/5
  "IW{2,1}(5,:)'"/1 -> dotprod5/1
  dotprod4/1 -> Mux/4
  "IW{2,1}(4,:)'"/1 -> dotprod4/1
  dotprod3/1 -> Mux/3
  "IW{2,1}(3,:)'"/1 -> dotprod3/1
  dotprod2/1 -> Mux/2
  "IW{2,1}(2,:)'"/1 -> dotprod2/1
  dotprod1/1 -> Mux/1
  "ad{2,1}"/1 -> dotprod10/2, dotprod9/2, dotprod8/2, dotprod7/2, dotprod6/2, dotprod5/2, dotprod4/2, dotprod3/2, dotprod2/2, dotprod1/2
  "IW{2,1}(1,:)'"/1 -> dotprod1/1

== system Current_torque_111/CNN/Layer 3/Delays 1 ==
  "p{3}" : Inport  PortDimensions=10
      mask Display: e = 0.06;c1 = [120 230 180]/255;c2 = ([120 230 180]+0)/(256+128);c3 = ([120 230 180]+128)/(256+128);patch([0 1 1 0],[0 0 1 1],c1);patch([0 1 1 1-e 1-e 0+e],[0 0 1 1-e 0+e 0+e],c2);patch([0 0 1 1-e 0+e 0+e],[0 1 1 1-e 1-e 0+e],c3);plot([0 1 1 0 0],[0 0 1 1 0]);
  mux : Mux  Inputs=1
      mask Display: e = 0.06;c1 = [120 150 230]/255;c2 = ([120 150 230]+0)/383;c3 = ([120 150 230]+128)/383;patch([0 1 1 0],[0 0 1 1],c1);patch([0 1 1 1-e 1-e 0+e],[0 0 1 1-e 0+e 0+e],c2);patch([0 0 1 1-e 0+e 0+e],[0 1 1 1-e 1-e 0+e],c3);plot([0 1 1 0 0],[0 0 1 1 0]);disp('Mux')
  "pd{3,2}" : Outport
      mask Display: e = 0.06;c1 = [120 230 180]/255;c2 = ([120 230 180]+0)/(256+128);c3 = ([120 230 180]+128)/(256+128);patch([0 1 1 0],[0 0 1 1],c1);patch([0 1 1 1-e 1-e 0+e],[0 0 1 1-e 0+e 0+e],c2);patch([0 0 1 1-e 0+e 0+e],[0 1 1 1-e 1-e 0+e],c3);plot([0 1 1 0 0],[0 0 1 1 0]);
  wires:
  mux/1 -> "pd{3,2}"/1
  "p{3}"/1 -> mux/1

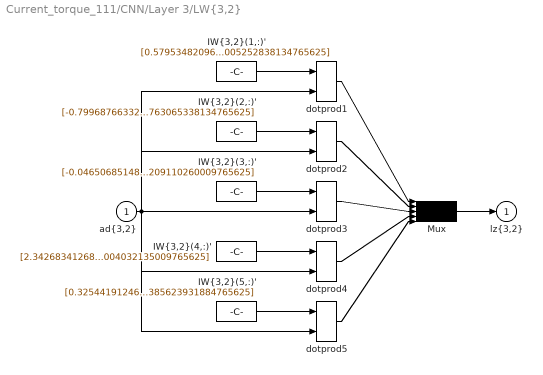
== system Current_torque_111/CNN/Layer 3/LW{3,2} ==
  "ad{3,2}" : Inport  PortDimensions=10
      mask Display: e = 0.06;c1 = [120 230 180]/255;c2 = ([120 230 180]+0)/(256+128);c3 = ([120 230 180]+128)/(256+128);patch([0 1 1 0],[0 0 1 1],c1);patch([0 1 1 1-e 1-e 0+e],[0 0 1 1-e 0+e 0+e],c2);patch([0 0 1 1-e 0+e 0+e],[0 1 1 1-e 1-e 0+e],c3);plot([0 1 1 0 0],[0 0 1 1 0]);
  "IW{3,2}(1,:)'" : Constant  Value=[0.579534820966327135494111644220538437366485595703125;-1.6471401977542547978572429201449267566204071044921875;0.59224090545491059334182182283257134258747100830078125;-2.57652253640741957241289128432981669902801513671875;1.8891463326443120873676662085927091538906097412109375;-1.729866707583904261724683237844146788120269775390625;0.03385849339439250815786408566054888069629669189453125;0.55820504375383295236900949021219275891780853271484375;1.503877580872905905806646842393092811107635498046875;0.99944940703688323058173637036816217005252838134765625]
      mask Display: e = 0.06;c1 = [120 150 230]/255;c2 = ([120 150 230]+0)/383;c3 = ([120 150 230]+128)/383;patch([0 1 1 0],[0 0 1 1],c1);patch([0 1 1 1-e 1-e 0+e],[0 0 1 1-e 0+e 0+e],c2);patch([0 0 1 1-e 0+e 0+e],[0 1 1 1-e 1-e 0+e],c3);plot([0 1 1 0 0],[0 0 1 1 0]);disp('weights');
  "IW{3,2}(2,:)'" : Constant  Value=[-0.79968766332044882716445499681867659091949462890625;0.08543614301456951831692521182048949413001537322998046875;0.363351870755110828437040026983595453202724456787109375;0.340427898913897963861785456174402497708797454833984375;0.1649368681912079248608193893232964910566806793212890625;-2.90266844181149519243945178459398448467254638671875;0.07769644058610793158070606523324386216700077056884765625;-0.1490642941243510433135810444582602940499782562255859375;-3.47456844003834053324908381910063326358795166015625;-0.443754685353645206280503998641506768763065338134765625]
      mask Display: e = 0.06;c1 = [120 150 230]/255;c2 = ([120 150 230]+0)/383;c3 = ([120 150 230]+128)/383;patch([0 1 1 0],[0 0 1 1],c1);patch([0 1 1 1-e 1-e 0+e],[0 0 1 1-e 0+e 0+e],c2);patch([0 0 1 1-e 0+e 0+e],[0 1 1 1-e 1-e 0+e],c3);plot([0 1 1 0 0],[0 0 1 1 0]);disp('weights');
  "IW{3,2}(3,:)'" : Constant  Value=[-0.046506851481905552014861626730635180138051509857177734375;-0.024926663352902035664104829493226134218275547027587890625;0.041353365415552963135770170310934190638363361358642578125;0.6981434610527530448820243691443465650081634521484375;-0.01289307520624781260021318729513950529508292675018310546875;2.1690703746946855545729704317636787891387939453125;0.031166433631050781405402716472963220439851284027099609375;-0.1160318971576430879810715168787282891571521759033203125;-0.75274770073975416639910918092937208712100982666015625;0.405406547543623096974130248781875707209110260009765625]
      mask Display: e = 0.06;c1 = [120 150 230]/255;c2 = ([120 150 230]+0)/383;c3 = ([120 150 230]+128)/383;patch([0 1 1 0],[0 0 1 1],c1);patch([0 1 1 1-e 1-e 0+e],[0 0 1 1-e 0+e 0+e],c2);patch([0 0 1 1-e 0+e 0+e],[0 1 1 1-e 1-e 0+e],c3);plot([0 1 1 0 0],[0 0 1 1 0]);disp('weights');
  "IW{3,2}(4,:)'" : Constant  Value=[2.34268341268654722853170824237167835235595703125;-1.9766342126418987579228314643842168152332305908203125;1.9791855275331833308172235774691216647624969482421875;-3.3357558333770942482487953384406864643096923828125;-1.811432488185079847653469187207520008087158203125;-1.3986380764302317469827130480553023517131805419921875;0.290092763400338904400399542282684706151485443115234375;0.226214277636696270423755095180240459740161895751953125;6.6289142375654446226462823688052594661712646484375;0.174483012576234719492873637136653997004032135009765625]
      mask Display: e = 0.06;c1 = [120 150 230]/255;c2 = ([120 150 230]+0)/383;c3 = ([120 150 230]+128)/383;patch([0 1 1 0],[0 0 1 1],c1);patch([0 1 1 1-e 1-e 0+e],[0 0 1 1-e 0+e 0+e],c2);patch([0 0 1 1-e 0+e 0+e],[0 1 1 1-e 1-e 0+e],c3);plot([0 1 1 0 0],[0 0 1 1 0]);disp('weights');
  "IW{3,2}(5,:)'" : Constant  Value=[0.325441912469127403451096824937849305570125579833984375;-0.87004318397808433349638335130293853580951690673828125;-0.887174187313692907963513789582066237926483154296875;1.7338064722101165227030605819891206920146942138671875;-0.1339278910887971019150199936120770871639251708984375;-0.055741399643950882702991833639316610060632228851318359375;-0.482479465056406431333613227252499200403690338134765625;-0.0652570046579753759719011441120528616011142730712890625;-1.8548192116593498202092860083212144672870635986328125;0.473535827635486461506530986298457719385623931884765625]
      mask Display: e = 0.06;c1 = [120 150 230]/255;c2 = ([120 150 230]+0)/383;c3 = ([120 150 230]+128)/383;patch([0 1 1 0],[0 0 1 1],c1);patch([0 1 1 1-e 1-e 0+e],[0 0 1 1-e 0+e 0+e],c2);patch([0 0 1 1-e 0+e 0+e],[0 1 1 1-e 1-e 0+e],c3);plot([0 1 1 0 0],[0 0 1 1 0]);disp('weights');
  Mux : Mux  Inputs=5
      mask Display: e = 0.06;c1 = [120 150 230]/255;c2 = ([120 150 230]+0)/383;c3 = ([120 150 230]+128)/383;patch([0 1 1 0],[0 0 1 1],c1);patch([0 1 1 1-e 1-e 0+e],[0 0 1 1-e 0+e 0+e],c2);patch([0 0 1 1-e 0+e 0+e],[0 1 1 1-e 1-e 0+e],c3);plot([0 1 1 0 0],[0 0 1 1 0]);disp('Mux');
  dotprod{1..5} (5 alike) : neural/Weight Functions/dotprod
  "lz{3,2}" : Outport
      mask Display: e = 0.06;c1 = [120 230 180]/255;c2 = ([120 230 180]+0)/(256+128);c3 = ([120 230 180]+128)/(256+128);patch([0 1 1 0],[0 0 1 1],c1);patch([0 1 1 1-e 1-e 0+e],[0 0 1 1-e 0+e 0+e],c2);patch([0 0 1 1-e 0+e 0+e],[0 1 1 1-e 1-e 0+e],c3);plot([0 1 1 0 0],[0 0 1 1 0]);
  wires:
  Mux/1 -> "lz{3,2}"/1
  dotprod5/1 -> Mux/5
  "IW{3,2}(5,:)'"/1 -> dotprod5/1
  dotprod4/1 -> Mux/4
  "IW{3,2}(4,:)'"/1 -> dotprod4/1
  dotprod3/1 -> Mux/3
  "IW{3,2}(3,:)'"/1 -> dotprod3/1
  dotprod2/1 -> Mux/2
  "IW{3,2}(2,:)'"/1 -> dotprod2/1
  dotprod1/1 -> Mux/1
  "ad{3,2}"/1 -> dotprod5/2, dotprod4/2, dotprod3/2, dotprod2/2, dotprod1/2
  "IW{3,2}(1,:)'"/1 -> dotprod1/1

== system Current_torque_111/CNN/Layer 4/Delays 1 ==
  "p{4}" : Inport  PortDimensions=5
      mask Display: e = 0.06;c1 = [120 230 180]/255;c2 = ([120 230 180]+0)/(256+128);c3 = ([120 230 180]+128)/(256+128);patch([0 1 1 0],[0 0 1 1],c1);patch([0 1 1 1-e 1-e 0+e],[0 0 1 1-e 0+e 0+e],c2);patch([0 0 1 1-e 0+e 0+e],[0 1 1 1-e 1-e 0+e],c3);plot([0 1 1 0 0],[0 0 1 1 0]);
  mux : Mux  Inputs=1
      mask Display: e = 0.06;c1 = [120 150 230]/255;c2 = ([120 150 230]+0)/383;c3 = ([120 150 230]+128)/383;patch([0 1 1 0],[0 0 1 1],c1);patch([0 1 1 1-e 1-e 0+e],[0 0 1 1-e 0+e 0+e],c2);patch([0 0 1 1-e 0+e 0+e],[0 1 1 1-e 1-e 0+e],c3);plot([0 1 1 0 0],[0 0 1 1 0]);disp('Mux')
  "pd{4,3}" : Outport
      mask Display: e = 0.06;c1 = [120 230 180]/255;c2 = ([120 230 180]+0)/(256+128);c3 = ([120 230 180]+128)/(256+128);patch([0 1 1 0],[0 0 1 1],c1);patch([0 1 1 1-e 1-e 0+e],[0 0 1 1-e 0+e 0+e],c2);patch([0 0 1 1-e 0+e 0+e],[0 1 1 1-e 1-e 0+e],c3);plot([0 1 1 0 0],[0 0 1 1 0]);
  wires:
  mux/1 -> "pd{4,3}"/1
  "p{4}"/1 -> mux/1

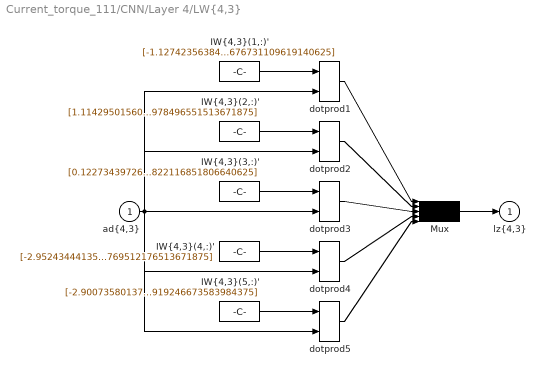
== system Current_torque_111/CNN/Layer 4/LW{4,3} ==
  "ad{4,3}" : Inport  PortDimensions=5
      mask Display: e = 0.06;c1 = [120 230 180]/255;c2 = ([120 230 180]+0)/(256+128);c3 = ([120 230 180]+128)/(256+128);patch([0 1 1 0],[0 0 1 1],c1);patch([0 1 1 1-e 1-e 0+e],[0 0 1 1-e 0+e 0+e],c2);patch([0 0 1 1-e 0+e 0+e],[0 1 1 1-e 1-e 0+e],c3);plot([0 1 1 0 0],[0 0 1 1 0]);
  "IW{4,3}(1,:)'" : Constant  Value=[-1.1274235638402598791429909397265873849391937255859375;-0.86074503416379244402634185462375171482563018798828125;-1.2962534158704113185223150139790959656238555908203125;0.07214585219906399782274775134283117949962615966796875;0.083867648934351779477225363734760321676731109619140625]
      mask Display: e = 0.06;c1 = [120 150 230]/255;c2 = ([120 150 230]+0)/383;c3 = ([120 150 230]+128)/383;patch([0 1 1 0],[0 0 1 1],c1);patch([0 1 1 1-e 1-e 0+e],[0 0 1 1-e 0+e 0+e],c2);patch([0 0 1 1-e 0+e 0+e],[0 1 1 1-e 1-e 0+e],c3);plot([0 1 1 0 0],[0 0 1 1 0]);disp('weights');
  "IW{4,3}(2,:)'" : Constant  Value=[1.1142950156050608345736918636248447000980377197265625;1.2489410049602132080082128595677204430103302001953125;2.167823196725443768428931434755213558673858642578125;0.191359525548705111663849720571306534111499786376953125;1.2325159658679865071206904758582822978496551513671875]
      mask Display: e = 0.06;c1 = [120 150 230]/255;c2 = ([120 150 230]+0)/383;c3 = ([120 150 230]+128)/383;patch([0 1 1 0],[0 0 1 1],c1);patch([0 1 1 1-e 1-e 0+e],[0 0 1 1-e 0+e 0+e],c2);patch([0 0 1 1-e 0+e 0+e],[0 1 1 1-e 1-e 0+e],c3);plot([0 1 1 0 0],[0 0 1 1 0]);disp('weights');
  "IW{4,3}(3,:)'" : Constant  Value=[0.12273439726345240774474376621583360247313976287841796875;-1.2981051101969758310161751069244928658008575439453125;0.054474747389556821275391484959982335567474365234375;0.099341070274438225684576764251687563955783843994140625;-1.101716966106467854302763953455723822116851806640625]
      mask Display: e = 0.06;c1 = [120 150 230]/255;c2 = ([120 150 230]+0)/383;c3 = ([120 150 230]+128)/383;patch([0 1 1 0],[0 0 1 1],c1);patch([0 1 1 1-e 1-e 0+e],[0 0 1 1-e 0+e 0+e],c2);patch([0 0 1 1-e 0+e 0+e],[0 1 1 1-e 1-e 0+e],c3);plot([0 1 1 0 0],[0 0 1 1 0]);disp('weights');
  "IW{4,3}(4,:)'" : Constant  Value=[-2.952434441356685201895970749319531023502349853515625;0.6065466786042603697381991878501139581203460693359375;1.6632055112426156195937210213742218911647796630859375;0.32970651193847577697937367702252231538295745849609375;0.1141520985841917024128377988745342008769512176513671875]
      mask Display: e = 0.06;c1 = [120 150 230]/255;c2 = ([120 150 230]+0)/383;c3 = ([120 150 230]+128)/383;patch([0 1 1 0],[0 0 1 1],c1);patch([0 1 1 1-e 1-e 0+e],[0 0 1 1-e 0+e 0+e],c2);patch([0 0 1 1-e 0+e 0+e],[0 1 1 1-e 1-e 0+e],c3);plot([0 1 1 0 0],[0 0 1 1 0]);disp('weights');
  "IW{4,3}(5,:)'" : Constant  Value=[-2.9007358013733579582549282349646091461181640625;0.59160149675123052670500101157813332974910736083984375;2.577612546155530370839414899819530546665191650390625;0.288077093930706684687947927159257233142852783203125;0.78833823185437468250569281735806725919246673583984375]
      mask Display: e = 0.06;c1 = [120 150 230]/255;c2 = ([120 150 230]+0)/383;c3 = ([120 150 230]+128)/383;patch([0 1 1 0],[0 0 1 1],c1);patch([0 1 1 1-e 1-e 0+e],[0 0 1 1-e 0+e 0+e],c2);patch([0 0 1 1-e 0+e 0+e],[0 1 1 1-e 1-e 0+e],c3);plot([0 1 1 0 0],[0 0 1 1 0]);disp('weights');
  Mux : Mux  Inputs=5
      mask Display: e = 0.06;c1 = [120 150 230]/255;c2 = ([120 150 230]+0)/383;c3 = ([120 150 230]+128)/383;patch([0 1 1 0],[0 0 1 1],c1);patch([0 1 1 1-e 1-e 0+e],[0 0 1 1-e 0+e 0+e],c2);patch([0 0 1 1-e 0+e 0+e],[0 1 1 1-e 1-e 0+e],c3);plot([0 1 1 0 0],[0 0 1 1 0]);disp('Mux');
  dotprod{1..5} (5 alike) : neural/Weight Functions/dotprod
  "lz{4,3}" : Outport
      mask Display: e = 0.06;c1 = [120 230 180]/255;c2 = ([120 230 180]+0)/(256+128);c3 = ([120 230 180]+128)/(256+128);patch([0 1 1 0],[0 0 1 1],c1);patch([0 1 1 1-e 1-e 0+e],[0 0 1 1-e 0+e 0+e],c2);patch([0 0 1 1-e 0+e 0+e],[0 1 1 1-e 1-e 0+e],c3);plot([0 1 1 0 0],[0 0 1 1 0]);
  wires:
  Mux/1 -> "lz{4,3}"/1
  dotprod5/1 -> Mux/5
  "IW{4,3}(5,:)'"/1 -> dotprod5/1
  dotprod4/1 -> Mux/4
  "IW{4,3}(4,:)'"/1 -> dotprod4/1
  dotprod3/1 -> Mux/3
  "IW{4,3}(3,:)'"/1 -> dotprod3/1
  dotprod2/1 -> Mux/2
  "IW{4,3}(2,:)'"/1 -> dotprod2/1
  dotprod1/1 -> Mux/1
  "ad{4,3}"/1 -> dotprod5/2, dotprod4/2, dotprod3/2, dotprod2/2, dotprod1/2
  "IW{4,3}(1,:)'"/1 -> dotprod1/1

== system Current_torque_111/CNN/Layer 5/Delays 1 ==
  "p{5}" : Inport  PortDimensions=5
      mask Display: e = 0.06;c1 = [120 230 180]/255;c2 = ([120 230 180]+0)/(256+128);c3 = ([120 230 180]+128)/(256+128);patch([0 1 1 0],[0 0 1 1],c1);patch([0 1 1 1-e 1-e 0+e],[0 0 1 1-e 0+e 0+e],c2);patch([0 0 1 1-e 0+e 0+e],[0 1 1 1-e 1-e 0+e],c3);plot([0 1 1 0 0],[0 0 1 1 0]);
  mux : Mux  Inputs=1
      mask Display: e = 0.06;c1 = [120 150 230]/255;c2 = ([120 150 230]+0)/383;c3 = ([120 150 230]+128)/383;patch([0 1 1 0],[0 0 1 1],c1);patch([0 1 1 1-e 1-e 0+e],[0 0 1 1-e 0+e 0+e],c2);patch([0 0 1 1-e 0+e 0+e],[0 1 1 1-e 1-e 0+e],c3);plot([0 1 1 0 0],[0 0 1 1 0]);disp('Mux')
  "pd{5,4}" : Outport
      mask Display: e = 0.06;c1 = [120 230 180]/255;c2 = ([120 230 180]+0)/(256+128);c3 = ([120 230 180]+128)/(256+128);patch([0 1 1 0],[0 0 1 1],c1);patch([0 1 1 1-e 1-e 0+e],[0 0 1 1-e 0+e 0+e],c2);patch([0 0 1 1-e 0+e 0+e],[0 1 1 1-e 1-e 0+e],c3);plot([0 1 1 0 0],[0 0 1 1 0]);
  wires:
  mux/1 -> "pd{5,4}"/1
  "p{5}"/1 -> mux/1

== system Current_torque_111/CNN/Layer 5/LW{5,4} ==
  "ad{5,4}" : Inport  PortDimensions=5
      mask Display: e = 0.06;c1 = [120 230 180]/255;c2 = ([120 230 180]+0)/(256+128);c3 = ([120 230 180]+128)/(256+128);patch([0 1 1 0],[0 0 1 1],c1);patch([0 1 1 1-e 1-e 0+e],[0 0 1 1-e 0+e 0+e],c2);patch([0 0 1 1-e 0+e 0+e],[0 1 1 1-e 1-e 0+e],c3);plot([0 1 1 0 0],[0 0 1 1 0]);
  "IW{5,4}(1,:)'" : Constant  Value=[-1.496059275884321859706460600136779248714447021484375;0.34734916354576939045983863252331502735614776611328125;-1.1870973210029156508227288213674910366535186767578125;-1.2153088318467251127685813116841018199920654296875;1.3671237018767843363065139783429913222789764404296875]
      mask Display: e = 0.06;c1 = [120 150 230]/255;c2 = ([120 150 230]+0)/383;c3 = ([120 150 230]+128)/383;patch([0 1 1 0],[0 0 1 1],c1);patch([0 1 1 1-e 1-e 0+e],[0 0 1 1-e 0+e 0+e],c2);patch([0 0 1 1-e 0+e 0+e],[0 1 1 1-e 1-e 0+e],c3);plot([0 1 1 0 0],[0 0 1 1 0]);disp('weights');
  Mux : Mux  Inputs=1
      mask Display: e = 0.06;c1 = [120 150 230]/255;c2 = ([120 150 230]+0)/383;c3 = ([120 150 230]+128)/383;patch([0 1 1 0],[0 0 1 1],c1);patch([0 1 1 1-e 1-e 0+e],[0 0 1 1-e 0+e 0+e],c2);patch([0 0 1 1-e 0+e 0+e],[0 1 1 1-e 1-e 0+e],c3);plot([0 1 1 0 0],[0 0 1 1 0]);disp('Mux');
  dotprod1 : neural/Weight Functions/dotprod
  "lz{5,4}" : Outport
      mask Display: e = 0.06;c1 = [120 230 180]/255;c2 = ([120 230 180]+0)/(256+128);c3 = ([120 230 180]+128)/(256+128);patch([0 1 1 0],[0 0 1 1],c1);patch([0 1 1 1-e 1-e 0+e],[0 0 1 1-e 0+e 0+e],c2);patch([0 0 1 1-e 0+e 0+e],[0 1 1 1-e 1-e 0+e],c3);plot([0 1 1 0 0],[0 0 1 1 0]);
  wires:
  Mux/1 -> "lz{5,4}"/1
  dotprod1/1 -> Mux/1
  "ad{5,4}"/1 -> dotprod1/2
  "IW{5,4}(1,:)'"/1 -> dotprod1/1

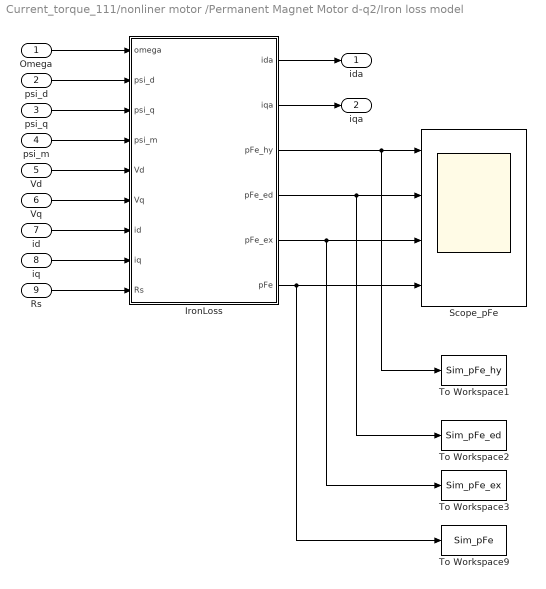
== system Current_torque_111/nonliner motor /Permanent Magnet Motor d-q2/Iron loss model ==
  Omega : Inport
  psi_d : Inport  Port=2
  psi_q : Inport  Port=3
  psi_m : Inport  Port=4
  Vd : Inport  Port=5
  Vq : Inport  Port=6
  id : Inport  Port=7
  iq : Inport  Port=8
  Rs : Inport  Port=9
  IronLoss : MATLAB Function  TreatAsAtomicUnit=on
  Scope_pFe : Scope  NumInputPorts=4
  To Workspace1 : ToWorkspace  VariableName=Sim_pFe_hy  SaveFormat=Structure With Time  SampleTime=-1
  To Workspace2 : ToWorkspace  VariableName=Sim_pFe_ed  SaveFormat=Structure With Time  SampleTime=-1
  To Workspace3 : ToWorkspace  VariableName=Sim_pFe_ex  SaveFormat=Structure With Time  SampleTime=-1
  To Workspace9 : ToWorkspace  VariableName=Sim_pFe  SaveFormat=Structure With Time  SampleTime=-1
  ida : Outport
  iqa : Outport  Port=2
  wires:
  IronLoss/5(pFe_ex) -> To Workspace3/1, Scope_pFe/3
  IronLoss/4(pFe_ed) -> To Workspace2/1, Scope_pFe/2
  IronLoss/3(pFe_hy) -> To Workspace1/1, Scope_pFe/1
  Rs/1 -> IronLoss/9(Rs)
  iq/1 -> IronLoss/8(iq)
  id/1 -> IronLoss/7(id)
  IronLoss/6(pFe) -> To Workspace9/1, Scope_pFe/4
  Vq/1 -> IronLoss/6(Vq)
  Vd/1 -> IronLoss/5(Vd)
  psi_m/1 -> IronLoss/4(psi_m)
  psi_q/1 -> IronLoss/3(psi_q)
  psi_d/1 -> IronLoss/2(psi_d)
  IronLoss/2(iqa) -> iqa/1
  IronLoss/1(ida) -> ida/1
  Omega/1 -> IronLoss/1(omega)
